simulink model "model"  (R2020b)
settings: Solver=VariableStepAuto  StartTime=0.0  StopTime=10.0  RelTol=1e-3
settings Model: Creator=SAGAR  LastModifiedBy=SAGAR

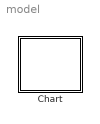
== system model ==
  Chart : Stateflow chart  TreatAsAtomicUnit=on

== stateflow chart model/Chart ==
  state got0
  state gpt_nickle
  state got_dime
  (default) -> got0
  got0 -> gpt_nickle [order 1] : [coin==1]{soda=0}
  gpt_nickle -> got0 [order 2] : [coin2==2]{soda=1}
  got_dime -> got0 [order 1] : [coin==1]{soda=1}
  got0 -> got_dime [order 2] : [coin==2]{soda=0}
  gpt_nickle -> got_dime [order 1] : [coin==1]{soda=0}
  got_dime -> gpt_nickle [order 2] : [coin==2]{soda=1}
